simulink model "sbvf_model_2019b_distributed"  (R2019b)
settings: Solver=VariableStepAuto  StartTime=0.0  StopTime=Tsim  RelTol=1e-3
undefined symbols (not defined in the file): A, A0, Ad, B, C, c, D, F, F_dist, Gdiag, k, K, K0, L_leader, std_dev, x0, x0_leader
libraries: dspindex x102, simulink x1
(part 2 of 2)

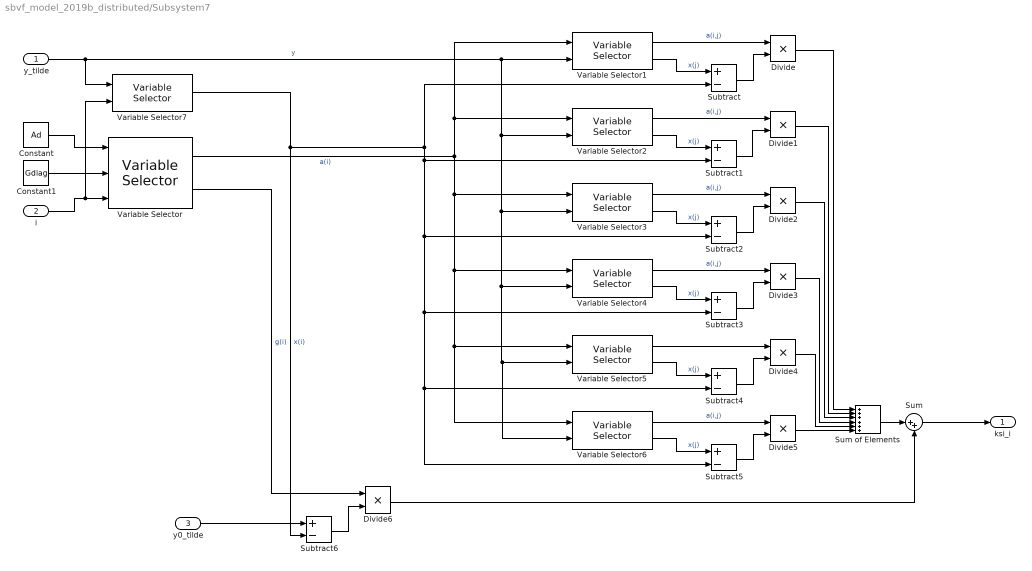
== system sbvf_model_2019b_distributed/Subsystem7 ==
  "y_tilde " : Inport
  i : Inport  Port=2
  "y0_tilde " : Inport  Port=3
  Constant : Constant  Value=Ad
  Constant1 : Constant  Value=Gdiag
  Divide{,1..6} (7 alike) : Product
  Subtract{,1..6} (7 alike) : Sum  Inputs=+-
  Sum : Sum  Inputs=|++
  Sum of Elements : Sum  Inputs=++++++
  Variable Selector : dspindex/Variable Selector  NumInputs=2  rowsOrCols=Rows  IdxMode=Variable  Elements=[1 3]  ZerOneIdxMode=One-based  errmode=Clip and Warn  FillMode=on  FillValues=0
  Variable Selector1 : dspindex/Variable Selector  NumInputs=2  rowsOrCols=Columns  IdxMode=Fixed  Elements=1  ZerOneIdxMode=One-based  errmode=Generate Error  FillMode=on  FillValues=0
  Variable Selector2 : dspindex/Variable Selector  NumInputs=2  rowsOrCols=Columns  IdxMode=Fixed  Elements=2  ZerOneIdxMode=One-based  errmode=Generate Error  FillMode=on  FillValues=0
  Variable Selector3 : dspindex/Variable Selector  NumInputs=2  rowsOrCols=Columns  IdxMode=Fixed  Elements=3  ZerOneIdxMode=One-based  errmode=Generate Error  FillMode=on  FillValues=0
  Variable Selector4 : dspindex/Variable Selector  NumInputs=2  rowsOrCols=Columns  IdxMode=Fixed  Elements=4  ZerOneIdxMode=One-based  errmode=Generate Error  FillMode=on  FillValues=0
  Variable Selector5 : dspindex/Variable Selector  NumInputs=2  rowsOrCols=Columns  IdxMode=Fixed  Elements=5  ZerOneIdxMode=One-based  errmode=Generate Error  FillMode=on  FillValues=0
  Variable Selector6 : dspindex/Variable Selector  NumInputs=2  rowsOrCols=Columns  IdxMode=Fixed  Elements=6  ZerOneIdxMode=One-based  errmode=Generate Error  FillMode=on  FillValues=0
  Variable Selector7 : dspindex/Variable Selector  NumInputs=1  rowsOrCols=Columns  IdxMode=Variable  Elements=1  ZerOneIdxMode=One-based  errmode=Generate Error  FillMode=on  FillValues=0
  ksi_i : Outport
  wires:
  Variable Selector/1 -> Variable Selector3/1, Variable Selector4/1, Variable Selector6/1, Variable Selector5/1, Variable Selector2/1, Variable Selector1/1  "a(i)"
  "y_tilde "/1 -> Variable Selector7/1, Variable Selector2/2, Variable Selector3/2, Variable Selector4/2, Variable Selector6/2, Variable Selector5/2, Variable Selector1/2  "y"
  Constant/1 -> Variable Selector/1
  i/1 -> Variable Selector7/2, Variable Selector/3
  Variable Selector1/1 -> Divide/1  "a(i,j)"
  Variable Selector1/2 -> Subtract/1  "x(j)"
  Subtract/1 -> Divide/2
  Variable Selector2/2 -> Subtract1/1  "x(j)"
  Variable Selector2/1 -> Divide1/1  "a(i,j)"
  Subtract1/1 -> Divide1/2
  Variable Selector3/1 -> Divide2/1  "a(i,j)"
  Variable Selector3/2 -> Subtract2/1  "x(j)"
  Subtract2/1 -> Divide2/2
  Variable Selector4/1 -> Divide3/1  "a(i,j)"
  Variable Selector4/2 -> Subtract3/1  "x(j)"
  Subtract3/1 -> Divide3/2
  Variable Selector5/2 -> Subtract4/1  "x(j)"
  Subtract4/1 -> Divide4/2
  Variable Selector5/1 -> Divide4/1
  Variable Selector6/1 -> Divide5/1  "a(i,j)"
  Variable Selector7/1 -> Subtract6/2, Subtract5/2, Subtract4/2, Subtract3/2, Subtract2/2, Subtract1/2, Subtract/2  "x(i)"
  Variable Selector6/2 -> Subtract5/1  "x(j)"
  Subtract5/1 -> Divide5/2
  Divide2/1 -> Sum of Elements/3
  Divide1/1 -> Sum of Elements/2
  Divide5/1 -> Sum of Elements/6
  Divide4/1 -> Sum of Elements/5
  Divide3/1 -> Sum of Elements/4
  Divide/1 -> Sum of Elements/1
  Variable Selector/2 -> Divide6/1  "g(i)"
  Subtract6/1 -> Divide6/2
  "y0_tilde "/1 -> Subtract6/1
  Divide6/1 -> Sum/2
  Sum of Elements/1 -> Sum/1
  Sum/1 -> ksi_i/1
  Constant1/1 -> Variable Selector/2

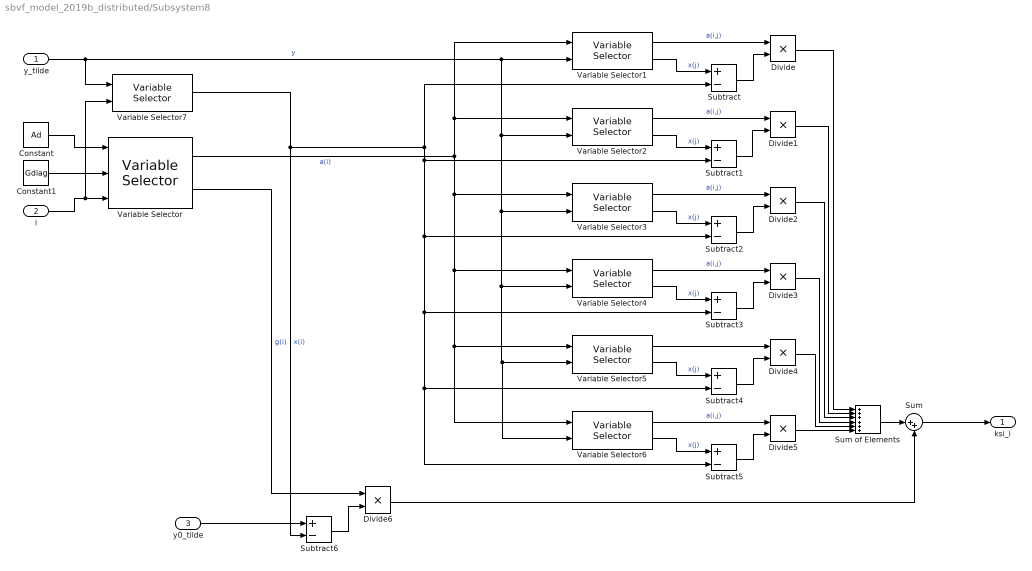
== system sbvf_model_2019b_distributed/Subsystem8 ==
  "y_tilde " : Inport
  i : Inport  Port=2
  "y0_tilde " : Inport  Port=3
  Constant : Constant  Value=Ad
  Constant1 : Constant  Value=Gdiag
  Divide{,1..6} (7 alike) : Product
  Subtract{,1..6} (7 alike) : Sum  Inputs=+-
  Sum : Sum  Inputs=|++
  Sum of Elements : Sum  Inputs=++++++
  Variable Selector : dspindex/Variable Selector  NumInputs=2  rowsOrCols=Rows  IdxMode=Variable  Elements=[1 3]  ZerOneIdxMode=One-based  errmode=Clip and Warn  FillMode=on  FillValues=0
  Variable Selector1 : dspindex/Variable Selector  NumInputs=2  rowsOrCols=Columns  IdxMode=Fixed  Elements=1  ZerOneIdxMode=One-based  errmode=Generate Error  FillMode=on  FillValues=0
  Variable Selector2 : dspindex/Variable Selector  NumInputs=2  rowsOrCols=Columns  IdxMode=Fixed  Elements=2  ZerOneIdxMode=One-based  errmode=Generate Error  FillMode=on  FillValues=0
  Variable Selector3 : dspindex/Variable Selector  NumInputs=2  rowsOrCols=Columns  IdxMode=Fixed  Elements=3  ZerOneIdxMode=One-based  errmode=Generate Error  FillMode=on  FillValues=0
  Variable Selector4 : dspindex/Variable Selector  NumInputs=2  rowsOrCols=Columns  IdxMode=Fixed  Elements=4  ZerOneIdxMode=One-based  errmode=Generate Error  FillMode=on  FillValues=0
  Variable Selector5 : dspindex/Variable Selector  NumInputs=2  rowsOrCols=Columns  IdxMode=Fixed  Elements=5  ZerOneIdxMode=One-based  errmode=Generate Error  FillMode=on  FillValues=0
  Variable Selector6 : dspindex/Variable Selector  NumInputs=2  rowsOrCols=Columns  IdxMode=Fixed  Elements=6  ZerOneIdxMode=One-based  errmode=Generate Error  FillMode=on  FillValues=0
  Variable Selector7 : dspindex/Variable Selector  NumInputs=1  rowsOrCols=Columns  IdxMode=Variable  Elements=1  ZerOneIdxMode=One-based  errmode=Generate Error  FillMode=on  FillValues=0
  ksi_i : Outport
  wires:
  Variable Selector/1 -> Variable Selector3/1, Variable Selector4/1, Variable Selector6/1, Variable Selector5/1, Variable Selector2/1, Variable Selector1/1  "a(i)"
  "y_tilde "/1 -> Variable Selector7/1, Variable Selector2/2, Variable Selector3/2, Variable Selector4/2, Variable Selector6/2, Variable Selector5/2, Variable Selector1/2  "y"
  Constant/1 -> Variable Selector/1
  i/1 -> Variable Selector7/2, Variable Selector/3
  Variable Selector1/1 -> Divide/1  "a(i,j)"
  Variable Selector1/2 -> Subtract/1  "x(j)"
  Subtract/1 -> Divide/2
  Variable Selector2/2 -> Subtract1/1  "x(j)"
  Variable Selector2/1 -> Divide1/1  "a(i,j)"
  Subtract1/1 -> Divide1/2
  Variable Selector3/1 -> Divide2/1  "a(i,j)"
  Variable Selector3/2 -> Subtract2/1  "x(j)"
  Subtract2/1 -> Divide2/2
  Variable Selector4/1 -> Divide3/1  "a(i,j)"
  Variable Selector4/2 -> Subtract3/1  "x(j)"
  Subtract3/1 -> Divide3/2
  Variable Selector5/2 -> Subtract4/1  "x(j)"
  Subtract4/1 -> Divide4/2
  Variable Selector5/1 -> Divide4/1
  Variable Selector6/1 -> Divide5/1  "a(i,j)"
  Variable Selector7/1 -> Subtract6/2, Subtract5/2, Subtract4/2, Subtract3/2, Subtract2/2, Subtract1/2, Subtract/2  "x(i)"
  Variable Selector6/2 -> Subtract5/1  "x(j)"
  Subtract5/1 -> Divide5/2
  Divide2/1 -> Sum of Elements/3
  Divide1/1 -> Sum of Elements/2
  Divide5/1 -> Sum of Elements/6
  Divide4/1 -> Sum of Elements/5
  Divide3/1 -> Sum of Elements/4
  Divide/1 -> Sum of Elements/1
  Variable Selector/2 -> Divide6/1  "g(i)"
  Subtract6/1 -> Divide6/2
  "y0_tilde "/1 -> Subtract6/1
  Divide6/1 -> Sum/2
  Sum of Elements/1 -> Sum/1
  Sum/1 -> ksi_i/1
  Constant1/1 -> Variable Selector/2

== system sbvf_model_2019b_distributed/Subsystem9 ==
  x : Inport
  i : Inport  Port=2
  x0 : Inport  Port=3
  Constant : Constant  Value=Ad
  Constant1 : Constant  Value=Gdiag
  Divide{,1..6} (7 alike) : Product
  Subtract{,1..6} (7 alike) : Sum  Inputs=+-
  Sum : Sum  Inputs=|++
  Sum of Elements : Sum  Inputs=++++++
  Variable Selector : dspindex/Variable Selector  NumInputs=2  rowsOrCols=Rows  IdxMode=Variable  Elements=[1 3]  ZerOneIdxMode=One-based  errmode=Clip and Warn  FillMode=on  FillValues=0
  Variable Selector1 : dspindex/Variable Selector  NumInputs=2  rowsOrCols=Columns  IdxMode=Fixed  Elements=1  ZerOneIdxMode=One-based  errmode=Generate Error  FillMode=on  FillValues=0
  Variable Selector2 : dspindex/Variable Selector  NumInputs=2  rowsOrCols=Columns  IdxMode=Fixed  Elements=2  ZerOneIdxMode=One-based  errmode=Generate Error  FillMode=on  FillValues=0
  Variable Selector3 : dspindex/Variable Selector  NumInputs=2  rowsOrCols=Columns  IdxMode=Fixed  Elements=3  ZerOneIdxMode=One-based  errmode=Generate Error  FillMode=on  FillValues=0
  Variable Selector4 : dspindex/Variable Selector  NumInputs=2  rowsOrCols=Columns  IdxMode=Fixed  Elements=4  ZerOneIdxMode=One-based  errmode=Generate Error  FillMode=on  FillValues=0
  Variable Selector5 : dspindex/Variable Selector  NumInputs=2  rowsOrCols=Columns  IdxMode=Fixed  Elements=5  ZerOneIdxMode=One-based  errmode=Generate Error  FillMode=on  FillValues=0
  Variable Selector6 : dspindex/Variable Selector  NumInputs=2  rowsOrCols=Columns  IdxMode=Fixed  Elements=6  ZerOneIdxMode=One-based  errmode=Generate Error  FillMode=on  FillValues=0
  Variable Selector7 : dspindex/Variable Selector  NumInputs=1  rowsOrCols=Columns  IdxMode=Variable  Elements=1  ZerOneIdxMode=One-based  errmode=Generate Error  FillMode=on  FillValues=0
  eps_i : Outport
  wires:
  Variable Selector/1 -> Variable Selector3/1, Variable Selector4/1, Variable Selector6/1, Variable Selector5/1, Variable Selector2/1, Variable Selector1/1  "a(i)"
  x/1 -> Variable Selector7/1, Variable Selector2/2, Variable Selector3/2, Variable Selector4/2, Variable Selector6/2, Variable Selector5/2, Variable Selector1/2  "x"
  Constant/1 -> Variable Selector/1
  i/1 -> Variable Selector7/2, Variable Selector/3
  Variable Selector1/1 -> Divide/1  "a(i,j)"
  Variable Selector1/2 -> Subtract/1  "x(j)"
  Subtract/1 -> Divide/2
  Variable Selector2/2 -> Subtract1/1  "x(j)"
  Variable Selector2/1 -> Divide1/1  "a(i,j)"
  Subtract1/1 -> Divide1/2
  Variable Selector3/1 -> Divide2/1  "a(i,j)"
  Variable Selector3/2 -> Subtract2/1  "x(j)"
  Subtract2/1 -> Divide2/2
  Variable Selector4/1 -> Divide3/1  "a(i,j)"
  Variable Selector4/2 -> Subtract3/1  "x(j)"
  Subtract3/1 -> Divide3/2
  Variable Selector5/2 -> Subtract4/1  "x(j)"
  Subtract4/1 -> Divide4/2
  Variable Selector5/1 -> Divide4/1
  Variable Selector6/1 -> Divide5/1  "a(i,j)"
  Variable Selector7/1 -> Subtract6/2, Subtract5/2, Subtract4/2, Subtract3/2, Subtract2/2, Subtract1/2, Subtract/2  "x(i)"
  Variable Selector6/2 -> Subtract5/1  "x(j)"
  Subtract5/1 -> Divide5/2
  Divide2/1 -> Sum of Elements/3
  Divide1/1 -> Sum of Elements/2
  Divide5/1 -> Sum of Elements/6
  Divide4/1 -> Sum of Elements/5
  Divide3/1 -> Sum of Elements/4
  Divide/1 -> Sum of Elements/1
  Variable Selector/2 -> Divide6/1  "g(i)"
  Subtract6/1 -> Divide6/2
  x0/1 -> Subtract6/1
  Divide6/1 -> Sum/2
  Sum of Elements/1 -> Sum/1
  Sum/1 -> eps_i/1
  Constant1/1 -> Variable Selector/2

== system sbvf_model_2019b_distributed/Ideal generator /Subsystem14 ==
  u : Inport
  "y " : Inport  Port=2
  Add1 : Sum  Inputs=+++
  Gain : Gain  Gain=c*L_leader  Multiplication=Matrix(K*u)
  Gain1 : Gain  Gain=B  Multiplication=Matrix(K*u)
  Gain2 : Gain  Gain=A0  Multiplication=Matrix(K*u)
  Gain3 : Gain  Gain=C  Multiplication=Matrix(K*u)
  Integrator : Integrator  InitialCondition=x0_leader
  Subtract : Sum  Inputs=-+
  x_hat : Outport
  wires:
  Gain2/1 -> Add1/3
  Gain/1 -> Add1/2
  Integrator/1 -> x_hat/1, Gain3/1, Gain2/1  "x_hat"
  Add1/1 -> Integrator/1  "x_hat_dot"
  u/1 -> Gain1/1
  Gain1/1 -> Add1/1
  "y "/1 -> Subtract/2
  Subtract/1 -> Gain/1
  Gain3/1 -> Subtract/1
